simulink library "inp"  (R2021b)
settings: Solver=VariableStepAuto  StartTime=0.0  StopTime=10.0  RelTol=1e-3
undefined symbols (not defined in the file): C_TASK_5MS_S, FALSE, KINP_AcoreReadyToSlp_flg_ovrdflg, KINP_AcoreReadyToSlp_flg_ovrdval, KINP_AllowMovThd_OTA_enum_ovrdflg, KINP_AllowMovThd_OTA_enum_ovrdval, KINP_APSAngleTarget_Deg_ovrdflg, KINP_APSAngleTarget_Deg_ovrdval, KINP_APSDecReq_mps2_ovrdflg, KINP_APSDecReq_mps2_ovrdval, KINP_APSDecReqA_flg_ovrdflg, KINP_APSDecReqA_flg_ovrdval, KINP_APSDFLL_cm_ovrdflg, KINP_APSDFLL_cm_ovrdval, KINP_APSDFLR_cm_ovrdflg, KINP_APSDFLR_cm_ovrdval, KINP_APSDRLL_cm_ovrdflg, KINP_APSDRLL_cm_ovrdval, KINP_APSDRLR_cm_ovrdflg, KINP_APSDRLR_cm_ovrdval, KINP_APSExitCondition_enum_ovrdflg, KINP_APSExitCondition_enum_ovrdval, KINP_APSHWVer_enum_ovrdflg, KINP_APSHWVer_enum_ovrdval, KINP_APSProgressPCT_pct_ovrdflg, KINP_APSProgressPCT_pct_ovrdval, KINP_APSReq_enum_ovrdflg, KINP_APSReq_enum_ovrdval, KINP_APSRQDisplay_enum_ovrdflg, KINP_APSRQDisplay_enum_ovrdval, KINP_APSRqEPASCtrl_flg_ovrdflg, KINP_APSRqEPASCtrl_flg_ovrdval, KINP_APSShiftPosnReq_enum_ovrdval, KINP_APSShiftPosnReq_enum_ovrflg, KINP_APSSpeedCMD_kph_ovrdval, KINP_APSSpeedCMD_kph_ovrflg, KINP_APSStaSystem_enum_ovrdflg, KINP_APSStaSystem_enum_ovrdval, KINP_APSSWVer_enum_ovrdflg, KINP_APSSWVer_enum_ovrdval, KINP_APSVMCReqA_flg_ovrdval, KINP_APSVMCReqA_flg_ovrflg, KINP_APSVRqEPASCtrl_flg_ovrdflg, KINP_APSVRqEPASCtrl_flg_ovrdval, KINP_AuxBattVolmV_mV_ovrdflg, KINP_AuxBattVolmV_mV_ovrdval, KINP_CAASSta_enum_ovrdflg, KINP_CAASSta_enum_ovrdval, KINP_CAASVMCReqA_flg_ovrdval, KINP_CAASVMCReqA_flg_ovrflg, KINP_Chime_enum_ovrdflg, KINP_Chime_enum_ovrdval, KINP_ClearDTCcmd_flg_ovrdflg, KINP_ClearDTCcmd_flg_ovrdval, KINP_EvccAplusPwrUpReq_flg_ovrdflg, KINP_EvccAplusPwrUpReq_flg_ovrdval, KINP_LFID_raw_ovrdval, KINP_LFID_raw_ovrflg, KINP_LRID_raw_ovrdval, KINP_MemOffsetAccX_raw16_ovrdflg ... (+118)
libraries: FVT_lib x595, hcu_lib x1
(part 16 of 27)

== system inp/INP/CAN3/SignalCheck/BMS3 ==
  BHAL_outputs : Inport
  inp_CanValid_bus : Inport  Port=2
  ACChrgCurrDis : FVT_lib/inp/can_signal_template  SystemSampleTime=-1  VariantActivationTime=update diagram  Latency=0  AutoFrameSizeCalculation=off
      link override defval: Value=KINP_ACChrgCurrDis_A_defval
      link override fftdec: Value=KINP_ACChrgCurrDis_A_fftdec
      link override fftinc: Value=KINP_ACChrgCurrDis_A_fftinc
      link override fftlim: Value=KINP_ACChrgCurrDis_A_fftlim
      link override invalid: Value=KINP_ACChrgCurrDis_A_invalid
      link override ovrdflg: Value=KINP_ACChrgCurrDis_A_ovrdflg
      link override ovrdval: Value=KINP_ACChrgCurrDis_A_ovrdval
      link override setvalid: Value=KINP_ACChrgCurrDis_A_setvalid
      link override srvcflg: Value=KINP_ACChrgCurrDis_A_srvcflg
      link override srvcval: Value=KINP_ACChrgCurrDis_A_srvcval
  HVBChrgPwr : FVT_lib/inp/can_signal_template  SystemSampleTime=-1  VariantActivationTime=update diagram  Latency=0  AutoFrameSizeCalculation=off
      link override defval: Value=KINP_HVBChrgPwr_kWh_defval
      link override fftdec: Value=KINP_HVBChrgPwr_kWh_fftdec
      link override fftinc: Value=KINP_HVBChrgPwr_kWh_fftinc
      link override fftlim: Value=KINP_HVBChrgPwr_kWh_fftlim
      link override invalid: Value=KINP_HVBChrgPwr_kWh_invalid
      link override ovrdflg: Value=KINP_HVBChrgPwr_kWh_ovrdflg
      link override ovrdval: Value=KINP_HVBChrgPwr_kWh_ovrdval
      link override setvalid: Value=KINP_HVBChrgPwr_kWh_setvalid
      link override srvcflg: Value=KINP_HVBChrgPwr_kWh_srvcflg
      link override srvcval: Value=KINP_HVBChrgPwr_kWh_srvcval
  HVBChrgPwrTotal : FVT_lib/inp/can_signal_template  SystemSampleTime=-1  VariantActivationTime=update diagram  Latency=0  AutoFrameSizeCalculation=off
      link override defval: Value=KINP_HVBChrgPwrTotal_kWh_defval
      link override fftdec: Value=KINP_HVBChrgPwrTotal_kWh_fftdec
      link override fftinc: Value=KINP_HVBChrgPwrTotal_kWh_fftinc
      link override fftlim: Value=KINP_HVBChrgPwrTotal_kWh_fftlim
      link override invalid: Value=KINP_HVBChrgPwrTotal_kWh_invalid
      link override ovrdflg: Value=KINP_HVBChrgPwrTotal_kWh_ovrdflg
      link override ovrdval: Value=KINP_HVBChrgPwrTotal_kWh_ovrdval
      link override setvalid: Value=KINP_HVBChrgPwrTotal_kWh_setvalid
      link override srvcflg: Value=KINP_HVBChrgPwrTotal_kWh_srvcflg
      link override srvcval: Value=KINP_HVBChrgPwrTotal_kWh_srvcval
  HVBDrvPwr : FVT_lib/inp/can_signal_template  SystemSampleTime=-1  VariantActivationTime=update diagram  Latency=0  AutoFrameSizeCalculation=off
      link override defval: Value=KINP_HVBDrvPwr_kWh_defval
      link override fftdec: Value=KINP_HVBDrvPwr_kWh_fftdec
      link override fftinc: Value=KINP_HVBDrvPwr_kWh_fftinc
      link override fftlim: Value=KINP_HVBDrvPwr_kWh_fftlim
      link override invalid: Value=KINP_HVBDrvPwr_kWh_invalid
      link override ovrdflg: Value=KINP_HVBDrvPwr_kWh_ovrdflg
      link override ovrdval: Value=KINP_HVBDrvPwr_kWh_ovrdval
      link override setvalid: Value=KINP_HVBDrvPwr_kWh_setvalid
      link override srvcflg: Value=KINP_HVBDrvPwr_kWh_srvcflg
      link override srvcval: Value=KINP_HVBDrvPwr_kWh_srvcval
  HVBDrvPwrTotal : FVT_lib/inp/can_signal_template  SystemSampleTime=-1  VariantActivationTime=update diagram  Latency=0  AutoFrameSizeCalculation=off
      link override defval: Value=KINP_HVBDrvPwrTotal_kWh_defval
      link override fftdec: Value=KINP_HVBDrvPwrTotal_kWh_fftdec
      link override fftinc: Value=KINP_HVBDrvPwrTotal_kWh_fftinc
      link override fftlim: Value=KINP_HVBDrvPwrTotal_kWh_fftlim
      link override invalid: Value=KINP_HVBDrvPwrTotal_kWh_invalid
      link override ovrdflg: Value=KINP_HVBDrvPwrTotal_kWh_ovrdflg
      link override ovrdval: Value=KINP_HVBDrvPwrTotal_kWh_ovrdval
      link override setvalid: Value=KINP_HVBDrvPwrTotal_kWh_setvalid
      link override srvcflg: Value=KINP_HVBDrvPwrTotal_kWh_srvcflg
      link override srvcval: Value=KINP_HVBDrvPwrTotal_kWh_srvcval
  HVBFullChrgPwr : FVT_lib/inp/can_signal_template  SystemSampleTime=-1  VariantActivationTime=update diagram  Latency=0  AutoFrameSizeCalculation=off
      link override defval: Value=KINP_HVBFullChrgPwr_kWh_defval
      link override fftdec: Value=KINP_HVBFullChrgPwr_kWh_fftdec
      link override fftinc: Value=KINP_HVBFullChrgPwr_kWh_fftinc
      link override fftlim: Value=KINP_HVBFullChrgPwr_kWh_fftlim
      link override invalid: Value=KINP_HVBFullChrgPwr_kWh_invalid
      link override ovrdflg: Value=KINP_HVBFullChrgPwr_kWh_ovrdflg
      link override ovrdval: Value=KINP_HVBFullChrgPwr_kWh_ovrdval
      link override setvalid: Value=KINP_HVBFullChrgPwr_kWh_setvalid
      link override srvcflg: Value=KINP_HVBFullChrgPwr_kWh_srvcflg
      link override srvcval: Value=KINP_HVBFullChrgPwr_kWh_srvcval
  HVBIsoImpedenceN : FVT_lib/inp/can_signal_template  SystemSampleTime=-1  VariantActivationTime=update diagram  Latency=0  AutoFrameSizeCalculation=off
      link override defval: Value=KINP_HVBIsoImpedenceN_Megaohm_defval
      link override fftdec: Value=KINP_HVBIsoImpedenceN_Megaohm_fftdec
      link override fftinc: Value=KINP_HVBIsoImpedenceN_Megaohm_fftinc
      link override fftlim: Value=KINP_HVBIsoImpedenceN_Megaohm_fftlim
      link override invalid: Value=KINP_HVBIsoImpedenceN_Megaohm_invalid
      link override ovrdflg: Value=KINP_HVBIsoImpedenceN_Megaohm_ovrdflg
      link override ovrdval: Value=KINP_HVBIsoImpedenceN_Megaohm_ovrdval
      link override setvalid: Value=KINP_HVBIsoImpedenceN_Megaohm_setvalid
      link override srvcflg: Value=KINP_HVBIsoImpedenceN_Megaohm_srvcflg
      link override srvcval: Value=KINP_HVBIsoImpedenceN_Megaohm_srvcval
  HVBIsoImpedenceP : FVT_lib/inp/can_signal_template  SystemSampleTime=-1  VariantActivationTime=update diagram  Latency=0  AutoFrameSizeCalculation=off
      link override defval: Value=KINP_HVBIsoImpedenceP_Megaohm_defval
      link override fftdec: Value=KINP_HVBIsoImpedenceP_Megaohm_fftdec
      link override fftinc: Value=KINP_HVBIsoImpedenceP_Megaohm_fftinc
      link override fftlim: Value=KINP_HVBIsoImpedenceP_Megaohm_fftlim
      link override invalid: Value=KINP_HVBIsoImpedenceP_Megaohm_invalid
      link override ovrdflg: Value=KINP_HVBIsoImpedenceP_Megaohm_ovrdflg
      link override ovrdval: Value=KINP_HVBIsoImpedenceP_Megaohm_ovrdval
      link override setvalid: Value=KINP_HVBIsoImpedenceP_Megaohm_setvalid
      link override srvcflg: Value=KINP_HVBIsoImpedenceP_Megaohm_srvcflg
      link override srvcval: Value=KINP_HVBIsoImpedenceP_Megaohm_srvcval
  HVBSOH : FVT_lib/inp/can_signal_template  SystemSampleTime=-1  VariantActivationTime=update diagram  Latency=0  AutoFrameSizeCalculation=off
      link override defval: Value=KINP_HVBSOH_pct_defval
      link override fftdec: Value=KINP_HVBSOH_pct_fftdec
      link override fftinc: Value=KINP_HVBSOH_pct_fftinc
      link override fftlim: Value=KINP_HVBSOH_pct_fftlim
      link override invalid: Value=KINP_HVBSOH_pct_invalid
      link override ovrdflg: Value=KINP_HVBSOH_pct_ovrdflg
      link override ovrdval: Value=KINP_HVBSOH_pct_ovrdval
      link override setvalid: Value=KINP_HVBSOH_pct_setvalid
      link override srvcflg: Value=KINP_HVBSOH_pct_srvcflg
      link override srvcval: Value=KINP_HVBSOH_pct_srvcval
  HVBattPackVolt : FVT_lib/inp/can_signal_template  SystemSampleTime=-1  VariantActivationTime=update diagram  Latency=0  AutoFrameSizeCalculation=off
      link override defval: Value=KINP_HVBattPackVolt_V_defval
      link override fftdec: Value=KINP_HVBattPackVolt_V_fftdec
      link override fftinc: Value=KINP_HVBattPackVolt_V_fftinc
      link override fftlim: Value=KINP_HVBattPackVolt_V_fftlim
      link override invalid: Value=KINP_HVBattPackVolt_V_invalid
      link override ovrdflg: Value=KINP_HVBattPackVolt_V_ovrdflg
      link override ovrdval: Value=KINP_HVBattPackVolt_V_ovrdval
      link override setvalid: Value=KINP_HVBattPackVolt_V_setvalid
      link override srvcflg: Value=KINP_HVBattPackVolt_V_srvcflg
      link override srvcval: Value=KINP_HVBattPackVolt_V_srvcval
  HVBattSOC : FVT_lib/inp/can_signal_template  SystemSampleTime=-1  VariantActivationTime=update diagram  Latency=0  AutoFrameSizeCalculation=off
      link override defval: Value=KINP_HVBattSOC_pct_defval
      link override fftdec: Value=KINP_HVBattSOC_pct_fftdec
      link override fftinc: Value=KINP_HVBattSOC_pct_fftinc
      link override fftlim: Value=KINP_HVBattSOC_pct_fftlim
      link override invalid: Value=KINP_HVBattSOC_pct_invalid
      link override ovrdflg: Value=KINP_HVBattSOC_pct_ovrdflg
      link override ovrdval: Value=KINP_HVBattSOC_pct_ovrdval
      link override setvalid: Value=KINP_HVBattSOC_pct_setvalid
      link override srvcflg: Value=KINP_HVBattSOC_pct_srvcflg
      link override srvcval: Value=KINP_HVBattSOC_pct_srvcval
  HVBattSOCDis : FVT_lib/inp/can_signal_template  SystemSampleTime=-1  VariantActivationTime=update diagram  Latency=0  AutoFrameSizeCalculation=off
      link override defval: Value=KINP_HVBattSOCDis_pct_defval
      link override fftdec: Value=KINP_HVBattSOCDis_pct_fftdec
      link override fftinc: Value=KINP_HVBattSOCDis_pct_fftinc
      link override fftlim: Value=KINP_HVBattSOCDis_pct_fftlim
      link override invalid: Value=KINP_HVBattSOCDis_pct_invalid
      link override ovrdflg: Value=KINP_HVBattSOCDis_pct_ovrdflg
      link override ovrdval: Value=KINP_HVBattSOCDis_pct_ovrdval
      link override setvalid: Value=KINP_HVBattSOCDis_pct_setvalid
      link override srvcflg: Value=KINP_HVBattSOCDis_pct_srvcflg
      link override srvcval: Value=KINP_HVBattSOCDis_pct_srvcval
  RemainChrgTime : FVT_lib/inp/can_signal_template  SystemSampleTime=-1  VariantActivationTime=update diagram  Latency=0  AutoFrameSizeCalculation=off
      link override defval: Value=KINP_RemainChrgTime_min_defval
      link override fftdec: Value=KINP_RemainChrgTime_min_fftdec
      link override fftinc: Value=KINP_RemainChrgTime_min_fftinc
      link override fftlim: Value=KINP_RemainChrgTime_min_fftlim
      link override invalid: Value=KINP_RemainChrgTime_min_invalid
      link override ovrdflg: Value=KINP_RemainChrgTime_min_ovrdflg
      link override ovrdval: Value=KINP_RemainChrgTime_min_ovrdval
      link override setvalid: Value=KINP_RemainChrgTime_min_setvalid
      link override srvcflg: Value=KINP_RemainChrgTime_min_srvcflg
      link override srvcval: Value=KINP_RemainChrgTime_min_srvcval
  Terminator_{1..13} (13 alike) : Terminator
  True_VHAL_ACChrgCurrDis_A : Constant  Value=TRUE  OutDataTypeStr=boolean
  True_VHAL_HVBChrgPwrTotal_kWh : Constant  Value=TRUE  OutDataTypeStr=boolean
  True_VHAL_HVBChrgPwr_kWh : Constant  Value=TRUE  OutDataTypeStr=boolean
  True_VHAL_HVBDrvPwrTotal_kWh : Constant  Value=TRUE  OutDataTypeStr=boolean
  True_VHAL_HVBDrvPwr_kWh : Constant  Value=TRUE  OutDataTypeStr=boolean
  True_VHAL_HVBFullChrgPwr_kWh : Constant  Value=TRUE  OutDataTypeStr=boolean
  True_VHAL_HVBIsoImpedenceN_Megaohm : Constant  Value=TRUE  OutDataTypeStr=boolean
  True_VHAL_HVBIsoImpedenceP_Megaohm : Constant  Value=TRUE  OutDataTypeStr=boolean
  True_VHAL_HVBSOH_pct : Constant  Value=TRUE  OutDataTypeStr=boolean
  True_VHAL_HVBattPackVolt_V : Constant  Value=TRUE  OutDataTypeStr=boolean
  True_VHAL_HVBattSOCDis_pct : Constant  Value=TRUE  OutDataTypeStr=boolean
  True_VHAL_HVBattSOC_pct : Constant  Value=TRUE  OutDataTypeStr=boolean
  True_VHAL_RemainChrgTime_min : Constant  Value=TRUE  OutDataTypeStr=boolean
  slr1_{1..13} (13 alike) : BusSelector  OutputSignals=VINP_CANMsgValidBMS3_flg
  slr_VHAL_ACChrgCurrDis_A : BusSelector  OutputSignals=VHAL_ACChrgCurrDis_A
  slr_VHAL_HVBChrgPwrTotal_kWh : BusSelector  OutputSignals=VHAL_HVBChrgPwrTotal_kWh
  slr_VHAL_HVBChrgPwr_kWh : BusSelector  OutputSignals=VHAL_HVBChrgPwr_kWh
  slr_VHAL_HVBDrvPwrTotal_kWh : BusSelector  OutputSignals=VHAL_HVBDrvPwrTotal_kWh
  slr_VHAL_HVBDrvPwr_kWh : BusSelector  OutputSignals=VHAL_HVBDrvPwr_kWh
  slr_VHAL_HVBFullChrgPwr_kWh : BusSelector  OutputSignals=VHAL_HVBFullChrgPwr_kWh
  slr_VHAL_HVBIsoImpedenceN_Megaohm : BusSelector  OutputSignals=VHAL_HVBIsoImpedenceN_Megaohm
  slr_VHAL_HVBIsoImpedenceP_Megaohm : BusSelector  OutputSignals=VHAL_HVBIsoImpedenceP_Megaohm
  slr_VHAL_HVBSOH_pct : BusSelector  OutputSignals=VHAL_HVBSOH_pct
  slr_VHAL_HVBattPackVolt_V : BusSelector  OutputSignals=VHAL_HVBattPackVolt_V
  slr_VHAL_HVBattSOCDis_pct : BusSelector  OutputSignals=VHAL_HVBattSOCDis_pct
  slr_VHAL_HVBattSOC_pct : BusSelector  OutputSignals=VHAL_HVBattSOC_pct
  slr_VHAL_RemainChrgTime_min : BusSelector  OutputSignals=VHAL_RemainChrgTime_min
  VINP_ACChrgCurrDis_A : Outport
  VINP_HVBChrgPwr_kWh : Outport  Port=2
  VINP_HVBChrgPwrTotal_kWh : Outport  Port=3
  VINP_HVBDrvPwr_kWh : Outport  Port=4
  VINP_HVBDrvPwrTotal_kWh : Outport  Port=5
  VINP_HVBFullChrgPwr_kWh : Outport  Port=6
  VINP_HVBIsoImpedenceN_Megaohm : Outport  Port=7
  VINP_HVBIsoImpedenceP_Megaohm : Outport  Port=8
  VINP_HVBSOH_pct : Outport  Port=9
  VINP_HVBattPackVolt_V : Outport  Port=10
  VINP_HVBattSOC_pct : Outport  Port=11
  VINP_HVBattSOCDis_pct : Outport  Port=12
  VINP_RemainChrgTime_min : Outport  Port=13
  wires:
  BHAL_outputs/1 -> [BHAL_outputs]
  inp_CanValid_bus/1 -> [inp_CanValid_bus]
  [BHAL_outputs] -> slr_VHAL_ACChrgCurrDis_A/1
  slr_VHAL_ACChrgCurrDis_A/1 -> ACChrgCurrDis/1  "<VHAL_ACChrgCurrDis_A>"
  True_VHAL_ACChrgCurrDis_A/1 -> ACChrgCurrDis/2
  [inp_CanValid_bus] -> slr1_1/1
  slr1_1/1 -> ACChrgCurrDis/3  "<VINP_CANMsgValidBMS3_flg>"
  ACChrgCurrDis/1 -> VINP_ACChrgCurrDis_A/1  "VINP_ACChrgCurrDis_A"
  ACChrgCurrDis/2 -> Terminator_1/1
  [BHAL_outputs] -> slr_VHAL_HVBChrgPwr_kWh/1
  slr_VHAL_HVBChrgPwr_kWh/1 -> HVBChrgPwr/1  "<VHAL_HVBChrgPwr_kWh>"
  True_VHAL_HVBChrgPwr_kWh/1 -> HVBChrgPwr/2
  [inp_CanValid_bus] -> slr1_2/1
  slr1_2/1 -> HVBChrgPwr/3  "<VINP_CANMsgValidBMS3_flg>"
  HVBChrgPwr/1 -> VINP_HVBChrgPwr_kWh/1  "VINP_HVBChrgPwr_kWh"
  HVBChrgPwr/2 -> Terminator_2/1
  [BHAL_outputs] -> slr_VHAL_HVBChrgPwrTotal_kWh/1
  slr_VHAL_HVBChrgPwrTotal_kWh/1 -> HVBChrgPwrTotal/1  "<VHAL_HVBChrgPwrTotal_kWh>"
  True_VHAL_HVBChrgPwrTotal_kWh/1 -> HVBChrgPwrTotal/2
  [inp_CanValid_bus] -> slr1_3/1
  slr1_3/1 -> HVBChrgPwrTotal/3  "<VINP_CANMsgValidBMS3_flg>"
  HVBChrgPwrTotal/1 -> VINP_HVBChrgPwrTotal_kWh/1  "VINP_HVBChrgPwrTotal_kWh"
  HVBChrgPwrTotal/2 -> Terminator_3/1
  [BHAL_outputs] -> slr_VHAL_HVBDrvPwr_kWh/1
  slr_VHAL_HVBDrvPwr_kWh/1 -> HVBDrvPwr/1  "<VHAL_HVBDrvPwr_kWh>"
  True_VHAL_HVBDrvPwr_kWh/1 -> HVBDrvPwr/2
  [inp_CanValid_bus] -> slr1_4/1
  slr1_4/1 -> HVBDrvPwr/3  "<VINP_CANMsgValidBMS3_flg>"
  HVBDrvPwr/1 -> VINP_HVBDrvPwr_kWh/1  "VINP_HVBDrvPwr_kWh"
  HVBDrvPwr/2 -> Terminator_4/1
  [BHAL_outputs] -> slr_VHAL_HVBDrvPwrTotal_kWh/1
  slr_VHAL_HVBDrvPwrTotal_kWh/1 -> HVBDrvPwrTotal/1  "<VHAL_HVBDrvPwrTotal_kWh>"
  True_VHAL_HVBDrvPwrTotal_kWh/1 -> HVBDrvPwrTotal/2
  [inp_CanValid_bus] -> slr1_5/1
  slr1_5/1 -> HVBDrvPwrTotal/3  "<VINP_CANMsgValidBMS3_flg>"
  HVBDrvPwrTotal/1 -> VINP_HVBDrvPwrTotal_kWh/1  "VINP_HVBDrvPwrTotal_kWh"
  HVBDrvPwrTotal/2 -> Terminator_5/1
  [BHAL_outputs] -> slr_VHAL_HVBFullChrgPwr_kWh/1
  slr_VHAL_HVBFullChrgPwr_kWh/1 -> HVBFullChrgPwr/1  "<VHAL_HVBFullChrgPwr_kWh>"
  True_VHAL_HVBFullChrgPwr_kWh/1 -> HVBFullChrgPwr/2
  [inp_CanValid_bus] -> slr1_6/1
  slr1_6/1 -> HVBFullChrgPwr/3  "<VINP_CANMsgValidBMS3_flg>"
  HVBFullChrgPwr/1 -> VINP_HVBFullChrgPwr_kWh/1  "VINP_HVBFullChrgPwr_kWh"
  HVBFullChrgPwr/2 -> Terminator_6/1
  [BHAL_outputs] -> slr_VHAL_HVBIsoImpedenceN_Megaohm/1
  slr_VHAL_HVBIsoImpedenceN_Megaohm/1 -> HVBIsoImpedenceN/1  "<VHAL_HVBIsoImpedenceN_Megaohm>"
  True_VHAL_HVBIsoImpedenceN_Megaohm/1 -> HVBIsoImpedenceN/2
  [inp_CanValid_bus] -> slr1_7/1
  slr1_7/1 -> HVBIsoImpedenceN/3  "<VINP_CANMsgValidBMS3_flg>"
  HVBIsoImpedenceN/1 -> VINP_HVBIsoImpedenceN_Megaohm/1  "VINP_HVBIsoImpedenceN_Megaohm"
  HVBIsoImpedenceN/2 -> Terminator_7/1
  [BHAL_outputs] -> slr_VHAL_HVBIsoImpedenceP_Megaohm/1
  slr_VHAL_HVBIsoImpedenceP_Megaohm/1 -> HVBIsoImpedenceP/1  "<VHAL_HVBIsoImpedenceP_Megaohm>"
  True_VHAL_HVBIsoImpedenceP_Megaohm/1 -> HVBIsoImpedenceP/2
  [inp_CanValid_bus] -> slr1_8/1
  slr1_8/1 -> HVBIsoImpedenceP/3  "<VINP_CANMsgValidBMS3_flg>"
  HVBIsoImpedenceP/1 -> VINP_HVBIsoImpedenceP_Megaohm/1  "VINP_HVBIsoImpedenceP_Megaohm"
  HVBIsoImpedenceP/2 -> Terminator_8/1
  [BHAL_outputs] -> slr_VHAL_HVBSOH_pct/1
  slr_VHAL_HVBSOH_pct/1 -> HVBSOH/1  "<VHAL_HVBSOH_pct>"
  True_VHAL_HVBSOH_pct/1 -> HVBSOH/2
  [inp_CanValid_bus] -> slr1_9/1
  slr1_9/1 -> HVBSOH/3  "<VINP_CANMsgValidBMS3_flg>"
  HVBSOH/1 -> VINP_HVBSOH_pct/1  "VINP_HVBSOH_pct"
  HVBSOH/2 -> Terminator_9/1
  [BHAL_outputs] -> slr_VHAL_HVBattPackVolt_V/1
  slr_VHAL_HVBattPackVolt_V/1 -> HVBattPackVolt/1  "<VHAL_HVBattPackVolt_V>"
  True_VHAL_HVBattPackVolt_V/1 -> HVBattPackVolt/2
  [inp_CanValid_bus] -> slr1_10/1
  slr1_10/1 -> HVBattPackVolt/3  "<VINP_CANMsgValidBMS3_flg>"
  HVBattPackVolt/1 -> VINP_HVBattPackVolt_V/1  "VINP_HVBattPackVolt_V"
  HVBattPackVolt/2 -> Terminator_10/1
  [BHAL_outputs] -> slr_VHAL_HVBattSOC_pct/1
  slr_VHAL_HVBattSOC_pct/1 -> HVBattSOC/1  "<VHAL_HVBattSOC_pct>"
  True_VHAL_HVBattSOC_pct/1 -> HVBattSOC/2
  [inp_CanValid_bus] -> slr1_11/1
  slr1_11/1 -> HVBattSOC/3  "<VINP_CANMsgValidBMS3_flg>"
  HVBattSOC/1 -> VINP_HVBattSOC_pct/1  "VINP_HVBattSOC_pct"
  HVBattSOC/2 -> Terminator_11/1
  [BHAL_outputs] -> slr_VHAL_HVBattSOCDis_pct/1
  slr_VHAL_HVBattSOCDis_pct/1 -> HVBattSOCDis/1  "<VHAL_HVBattSOCDis_pct>"
  True_VHAL_HVBattSOCDis_pct/1 -> HVBattSOCDis/2
  [inp_CanValid_bus] -> slr1_12/1
  slr1_12/1 -> HVBattSOCDis/3  "<VINP_CANMsgValidBMS3_flg>"
  HVBattSOCDis/1 -> VINP_HVBattSOCDis_pct/1  "VINP_HVBattSOCDis_pct"
  HVBattSOCDis/2 -> Terminator_12/1
  [BHAL_outputs] -> slr_VHAL_RemainChrgTime_min/1
  slr_VHAL_RemainChrgTime_min/1 -> RemainChrgTime/1  "<VHAL_RemainChrgTime_min>"
  True_VHAL_RemainChrgTime_min/1 -> RemainChrgTime/2
  [inp_CanValid_bus] -> slr1_13/1
  slr1_13/1 -> RemainChrgTime/3  "<VINP_CANMsgValidBMS3_flg>"
  RemainChrgTime/1 -> VINP_RemainChrgTime_min/1  "VINP_RemainChrgTime_min"
  RemainChrgTime/2 -> Terminator_13/1

== system inp/INP/CAN3/SignalCheck/BMS4 ==
  BHAL_outputs : Inport
  inp_CanValid_bus : Inport  Port=2
  CellTempAvg : FVT_lib/inp/can_signal_template  SystemSampleTime=-1  VariantActivationTime=update diagram  Latency=0  AutoFrameSizeCalculation=off
      link override defval: Value=KINP_CellTempAvg_C_defval
      link override fftdec: Value=KINP_CellTempAvg_C_fftdec
      link override fftinc: Value=KINP_CellTempAvg_C_fftinc
      link override fftlim: Value=KINP_CellTempAvg_C_fftlim
      link override invalid: Value=KINP_CellTempAvg_C_invalid
      link override ovrdflg: Value=KINP_CellTempAvg_C_ovrdflg
      link override ovrdval: Value=KINP_CellTempAvg_C_ovrdval
      link override setvalid: Value=KINP_CellTempAvg_C_setvalid
      link override srvcflg: Value=KINP_CellTempAvg_C_srvcflg
      link override srvcval: Value=KINP_CellTempAvg_C_srvcval
  HVBCellVoltMax : FVT_lib/inp/can_signal_template  SystemSampleTime=-1  VariantActivationTime=update diagram  Latency=0  AutoFrameSizeCalculation=off
      link override defval: Value=KINP_HVBCellVoltMax_mV_defval
      link override fftdec: Value=KINP_HVBCellVoltMax_mV_fftdec
      link override fftinc: Value=KINP_HVBCellVoltMax_mV_fftinc
      link override fftlim: Value=KINP_HVBCellVoltMax_mV_fftlim
      link override invalid: Value=KINP_HVBCellVoltMax_mV_invalid
      link override ovrdflg: Value=KINP_HVBCellVoltMax_mV_ovrdflg
      link override ovrdval: Value=KINP_HVBCellVoltMax_mV_ovrdval
      link override setvalid: Value=KINP_HVBCellVoltMax_mV_setvalid
      link override srvcflg: Value=KINP_HVBCellVoltMax_mV_srvcflg
      link override srvcval: Value=KINP_HVBCellVoltMax_mV_srvcval
  HVBCellVoltMin : FVT_lib/inp/can_signal_template  SystemSampleTime=-1  VariantActivationTime=update diagram  Latency=0  AutoFrameSizeCalculation=off
      link override defval: Value=KINP_HVBCellVoltMin_mV_defval
      link override fftdec: Value=KINP_HVBCellVoltMin_mV_fftdec
      link override fftinc: Value=KINP_HVBCellVoltMin_mV_fftinc
      link override fftlim: Value=KINP_HVBCellVoltMin_mV_fftlim
      link override invalid: Value=KINP_HVBCellVoltMin_mV_invalid
      link override ovrdflg: Value=KINP_HVBCellVoltMin_mV_ovrdflg
      link override ovrdval: Value=KINP_HVBCellVoltMin_mV_ovrdval
      link override setvalid: Value=KINP_HVBCellVoltMin_mV_setvalid
      link override srvcflg: Value=KINP_HVBCellVoltMin_mV_srvcflg
      link override srvcval: Value=KINP_HVBCellVoltMin_mV_srvcval
  HVBMTempMax : FVT_lib/inp/can_signal_template  SystemSampleTime=-1  VariantActivationTime=update diagram  Latency=0  AutoFrameSizeCalculation=off
      link override defval: Value=KINP_HVBMTempMax_C_defval
      link override fftdec: Value=KINP_HVBMTempMax_C_fftdec
      link override fftinc: Value=KINP_HVBMTempMax_C_fftinc
      link override fftlim: Value=KINP_HVBMTempMax_C_fftlim
      link override invalid: Value=KINP_HVBMTempMax_C_invalid
      link override ovrdflg: Value=KINP_HVBMTempMax_C_ovrdflg
      link override ovrdval: Value=KINP_HVBMTempMax_C_ovrdval
      link override setvalid: Value=KINP_HVBMTempMax_C_setvalid
      link override srvcflg: Value=KINP_HVBMTempMax_C_srvcflg
      link override srvcval: Value=KINP_HVBMTempMax_C_srvcval
  HVBMTempMin : FVT_lib/inp/can_signal_template  SystemSampleTime=-1  VariantActivationTime=update diagram  Latency=0  AutoFrameSizeCalculation=off
      link override defval: Value=KINP_HVBMTempMin_C_defval
      link override fftdec: Value=KINP_HVBMTempMin_C_fftdec
      link override fftinc: Value=KINP_HVBMTempMin_C_fftinc
      link override fftlim: Value=KINP_HVBMTempMin_C_fftlim
      link override invalid: Value=KINP_HVBMTempMin_C_invalid
      link override ovrdflg: Value=KINP_HVBMTempMin_C_ovrdflg
      link override ovrdval: Value=KINP_HVBMTempMin_C_ovrdval
      link override setvalid: Value=KINP_HVBMTempMin_C_setvalid
      link override srvcflg: Value=KINP_HVBMTempMin_C_srvcflg
      link override srvcval: Value=KINP_HVBMTempMin_C_srvcval
  MaxCellTempNum : FVT_lib/inp/can_signal_template  SystemSampleTime=-1  VariantActivationTime=update diagram  Latency=0  AutoFrameSizeCalculation=off
      link override defval: Value=KINP_MaxCellTempNum_enum_defval
      link override fftdec: Value=KINP_MaxCellTempNum_enum_fftdec
      link override fftinc: Value=KINP_MaxCellTempNum_enum_fftinc
      link override fftlim: Value=KINP_MaxCellTempNum_enum_fftlim
      link override invalid: Value=KINP_MaxCellTempNum_enum_invalid
      link override ovrdflg: Value=KINP_MaxCellTempNum_enum_ovrdflg
      link override ovrdval: Value=KINP_MaxCellTempNum_enum_ovrdval
      link override setvalid: Value=KINP_MaxCellTempNum_enum_setvalid
      link override srvcflg: Value=KINP_MaxCellTempNum_enum_srvcflg
      link override srvcval: Value=KINP_MaxCellTempNum_enum_srvcval
  MaxCellVoltNum : FVT_lib/inp/can_signal_template  SystemSampleTime=-1  VariantActivationTime=update diagram  Latency=0  AutoFrameSizeCalculation=off
      link override defval: Value=KINP_MaxCellVoltNum_enum_defval
      link override fftdec: Value=KINP_MaxCellVoltNum_enum_fftdec
      link override fftinc: Value=KINP_MaxCellVoltNum_enum_fftinc
      link override fftlim: Value=KINP_MaxCellVoltNum_enum_fftlim
      link override invalid: Value=KINP_MaxCellVoltNum_enum_invalid
      link override ovrdflg: Value=KINP_MaxCellVoltNum_enum_ovrdflg
      link override ovrdval: Value=KINP_MaxCellVoltNum_enum_ovrdval
      link override setvalid: Value=KINP_MaxCellVoltNum_enum_setvalid
      link override srvcflg: Value=KINP_MaxCellVoltNum_enum_srvcflg
      link override srvcval: Value=KINP_MaxCellVoltNum_enum_srvcval
  MinCellTempNum : FVT_lib/inp/can_signal_template  SystemSampleTime=-1  VariantActivationTime=update diagram  Latency=0  AutoFrameSizeCalculation=off
      link override defval: Value=KINP_MinCellTempNum_enum_defval
      link override fftdec: Value=KINP_MinCellTempNum_enum_fftdec
      link override fftinc: Value=KINP_MinCellTempNum_enum_fftinc
      link override fftlim: Value=KINP_MinCellTempNum_enum_fftlim
      link override invalid: Value=KINP_MinCellTempNum_enum_invalid
      link override ovrdflg: Value=KINP_MinCellTempNum_enum_ovrdflg
      link override ovrdval: Value=KINP_MinCellTempNum_enum_ovrdval
      link override setvalid: Value=KINP_MinCellTempNum_enum_setvalid
      link override srvcflg: Value=KINP_MinCellTempNum_enum_srvcflg
      link override srvcval: Value=KINP_MinCellTempNum_enum_srvcval
  MinCellVoltNum : FVT_lib/inp/can_signal_template  SystemSampleTime=-1  VariantActivationTime=update diagram  Latency=0  AutoFrameSizeCalculation=off
      link override defval: Value=KINP_MinCellVoltNum_enum_defval
      link override fftdec: Value=KINP_MinCellVoltNum_enum_fftdec
      link override fftinc: Value=KINP_MinCellVoltNum_enum_fftinc
      link override fftlim: Value=KINP_MinCellVoltNum_enum_fftlim
      link override invalid: Value=KINP_MinCellVoltNum_enum_invalid
      link override ovrdflg: Value=KINP_MinCellVoltNum_enum_ovrdflg
      link override ovrdval: Value=KINP_MinCellVoltNum_enum_ovrdval
      link override setvalid: Value=KINP_MinCellVoltNum_enum_setvalid
      link override srvcflg: Value=KINP_MinCellVoltNum_enum_srvcflg
      link override srvcval: Value=KINP_MinCellVoltNum_enum_srvcval
  Terminator_{1..9} (9 alike) : Terminator
  True_VHAL_CellTempAvg_C : Constant  Value=TRUE  OutDataTypeStr=boolean
  True_VHAL_HVBCellVoltMax_mV : Constant  Value=TRUE  OutDataTypeStr=boolean
  True_VHAL_HVBCellVoltMin_mV : Constant  Value=TRUE  OutDataTypeStr=boolean
  True_VHAL_HVBMTempMax_C : Constant  Value=TRUE  OutDataTypeStr=boolean
  True_VHAL_HVBMTempMin_C : Constant  Value=TRUE  OutDataTypeStr=boolean
  True_VHAL_MaxCellTempNum_enum : Constant  Value=TRUE  OutDataTypeStr=boolean
  True_VHAL_MaxCellVoltNum_enum : Constant  Value=TRUE  OutDataTypeStr=boolean
  True_VHAL_MinCellTempNum_enum : Constant  Value=TRUE  OutDataTypeStr=boolean
  True_VHAL_MinCellVoltNum_enum : Constant  Value=TRUE  OutDataTypeStr=boolean
  slr1_{1..9} (9 alike) : BusSelector  OutputSignals=VINP_CANMsgValidBMS4_flg
  slr_VHAL_CellTempAvg_C : BusSelector  OutputSignals=VHAL_CellTempAvg_C
  slr_VHAL_HVBCellVoltMax_mV : BusSelector  OutputSignals=VHAL_HVBCellVoltMax_mV
  slr_VHAL_HVBCellVoltMin_mV : BusSelector  OutputSignals=VHAL_HVBCellVoltMin_mV
  slr_VHAL_HVBMTempMax_C : BusSelector  OutputSignals=VHAL_HVBMTempMax_C
  slr_VHAL_HVBMTempMin_C : BusSelector  OutputSignals=VHAL_HVBMTempMin_C
  slr_VHAL_MaxCellTempNum_enum : BusSelector  OutputSignals=VHAL_MaxCellTempNum_enum
  slr_VHAL_MaxCellVoltNum_enum : BusSelector  OutputSignals=VHAL_MaxCellVoltNum_enum
  slr_VHAL_MinCellTempNum_enum : BusSelector  OutputSignals=VHAL_MinCellTempNum_enum
  slr_VHAL_MinCellVoltNum_enum : BusSelector  OutputSignals=VHAL_MinCellVoltNum_enum
  VINP_CellTempAvg_C : Outport
  VINP_HVBCellVoltMax_mV : Outport  Port=2
  VINP_HVBCellVoltMin_mV : Outport  Port=3
  VINP_HVBMTempMax_C : Outport  Port=4
  VINP_HVBMTempMin_C : Outport  Port=5
  VINP_MaxCellTempNum_enum : Outport  Port=6
  VINP_MaxCellVoltNum_enum : Outport  Port=7
  VINP_MinCellTempNum_enum : Outport  Port=8
  VINP_MinCellVoltNum_enum : Outport  Port=9
  wires:
  BHAL_outputs/1 -> [BHAL_outputs]
  inp_CanValid_bus/1 -> [inp_CanValid_bus]
  [BHAL_outputs] -> slr_VHAL_CellTempAvg_C/1
  slr_VHAL_CellTempAvg_C/1 -> CellTempAvg/1  "<VHAL_CellTempAvg_C>"
  True_VHAL_CellTempAvg_C/1 -> CellTempAvg/2
  [inp_CanValid_bus] -> slr1_1/1
  slr1_1/1 -> CellTempAvg/3  "<VINP_CANMsgValidBMS4_flg>"
  CellTempAvg/1 -> VINP_CellTempAvg_C/1  "VINP_CellTempAvg_C"
  CellTempAvg/2 -> Terminator_1/1
  [BHAL_outputs] -> slr_VHAL_HVBCellVoltMax_mV/1
  slr_VHAL_HVBCellVoltMax_mV/1 -> HVBCellVoltMax/1  "<VHAL_HVBCellVoltMax_mV>"
  True_VHAL_HVBCellVoltMax_mV/1 -> HVBCellVoltMax/2
  [inp_CanValid_bus] -> slr1_2/1
  slr1_2/1 -> HVBCellVoltMax/3  "<VINP_CANMsgValidBMS4_flg>"
  HVBCellVoltMax/1 -> VINP_HVBCellVoltMax_mV/1  "VINP_HVBCellVoltMax_mV"
  HVBCellVoltMax/2 -> Terminator_2/1
  [BHAL_outputs] -> slr_VHAL_HVBCellVoltMin_mV/1
  slr_VHAL_HVBCellVoltMin_mV/1 -> HVBCellVoltMin/1  "<VHAL_HVBCellVoltMin_mV>"
  True_VHAL_HVBCellVoltMin_mV/1 -> HVBCellVoltMin/2
  [inp_CanValid_bus] -> slr1_3/1
  slr1_3/1 -> HVBCellVoltMin/3  "<VINP_CANMsgValidBMS4_flg>"
  HVBCellVoltMin/1 -> VINP_HVBCellVoltMin_mV/1  "VINP_HVBCellVoltMin_mV"
  HVBCellVoltMin/2 -> Terminator_3/1
  [BHAL_outputs] -> slr_VHAL_HVBMTempMax_C/1
  slr_VHAL_HVBMTempMax_C/1 -> HVBMTempMax/1  "<VHAL_HVBMTempMax_C>"
  True_VHAL_HVBMTempMax_C/1 -> HVBMTempMax/2
  [inp_CanValid_bus] -> slr1_4/1
  slr1_4/1 -> HVBMTempMax/3  "<VINP_CANMsgValidBMS4_flg>"
  HVBMTempMax/1 -> VINP_HVBMTempMax_C/1  "VINP_HVBMTempMax_C"
  HVBMTempMax/2 -> Terminator_4/1
  [BHAL_outputs] -> slr_VHAL_HVBMTempMin_C/1
  slr_VHAL_HVBMTempMin_C/1 -> HVBMTempMin/1  "<VHAL_HVBMTempMin_C>"
  True_VHAL_HVBMTempMin_C/1 -> HVBMTempMin/2
  [inp_CanValid_bus] -> slr1_5/1
  slr1_5/1 -> HVBMTempMin/3  "<VINP_CANMsgValidBMS4_flg>"
  HVBMTempMin/1 -> VINP_HVBMTempMin_C/1  "VINP_HVBMTempMin_C"
  HVBMTempMin/2 -> Terminator_5/1
  [BHAL_outputs] -> slr_VHAL_MaxCellTempNum_enum/1
  slr_VHAL_MaxCellTempNum_enum/1 -> MaxCellTempNum/1  "<VHAL_MaxCellTempNum_enum>"
  True_VHAL_MaxCellTempNum_enum/1 -> MaxCellTempNum/2
  [inp_CanValid_bus] -> slr1_6/1
  slr1_6/1 -> MaxCellTempNum/3  "<VINP_CANMsgValidBMS4_flg>"
  MaxCellTempNum/1 -> VINP_MaxCellTempNum_enum/1  "VINP_MaxCellTempNum_enum"
  MaxCellTempNum/2 -> Terminator_6/1
  [BHAL_outputs] -> slr_VHAL_MaxCellVoltNum_enum/1
  slr_VHAL_MaxCellVoltNum_enum/1 -> MaxCellVoltNum/1  "<VHAL_MaxCellVoltNum_enum>"
  True_VHAL_MaxCellVoltNum_enum/1 -> MaxCellVoltNum/2
  [inp_CanValid_bus] -> slr1_7/1
  slr1_7/1 -> MaxCellVoltNum/3  "<VINP_CANMsgValidBMS4_flg>"
  MaxCellVoltNum/1 -> VINP_MaxCellVoltNum_enum/1  "VINP_MaxCellVoltNum_enum"
  MaxCellVoltNum/2 -> Terminator_7/1
  [BHAL_outputs] -> slr_VHAL_MinCellTempNum_enum/1
  slr_VHAL_MinCellTempNum_enum/1 -> MinCellTempNum/1  "<VHAL_MinCellTempNum_enum>"
  True_VHAL_MinCellTempNum_enum/1 -> MinCellTempNum/2
  [inp_CanValid_bus] -> slr1_8/1
  slr1_8/1 -> MinCellTempNum/3  "<VINP_CANMsgValidBMS4_flg>"
  MinCellTempNum/1 -> VINP_MinCellTempNum_enum/1  "VINP_MinCellTempNum_enum"
  MinCellTempNum/2 -> Terminator_8/1
  [BHAL_outputs] -> slr_VHAL_MinCellVoltNum_enum/1
  slr_VHAL_MinCellVoltNum_enum/1 -> MinCellVoltNum/1  "<VHAL_MinCellVoltNum_enum>"
  True_VHAL_MinCellVoltNum_enum/1 -> MinCellVoltNum/2
  [inp_CanValid_bus] -> slr1_9/1
  slr1_9/1 -> MinCellVoltNum/3  "<VINP_CANMsgValidBMS4_flg>"
  MinCellVoltNum/1 -> VINP_MinCellVoltNum_enum/1  "VINP_MinCellVoltNum_enum"
  MinCellVoltNum/2 -> Terminator_9/1
